simulink model "scheme1_analysis_aw"  (R2019b)
settings: Solver=ode4  StartTime=0.0  StopTime=30  FixedStep=0.1  RelTol=1e-3
values from neighbouring files (symbols this model uses):
  Kaw = 10    [solution.m]
  Kd = K(3)    [solution.m]
  Ki = K(1)    [solution.m]
  Kp = K(2)    [solution.m]
settings Model: Creator=biannic  LastModifiedBy=biannic
settings DataIOCC: ReturnWorkspaceOutputs=off

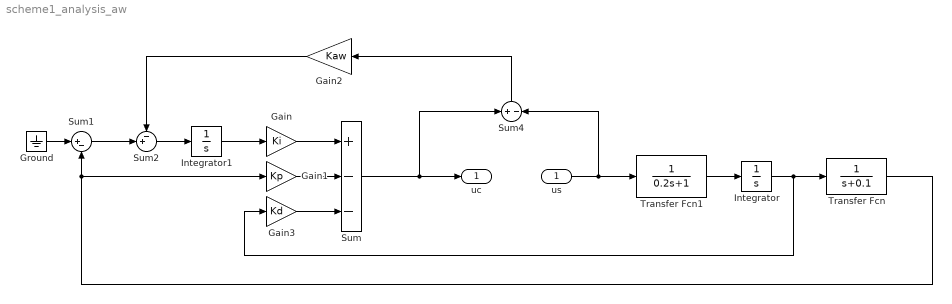
== system scheme1_analysis_aw ==
  us : Inport
  Gain : Gain  Gain=Ki
  Gain1 : Gain  Gain=Kp
  Gain2 : Gain  Gain=Kaw
  Gain3 : Gain  Gain=Kd
  Ground : Ground
  Integrator : Integrator
  Integrator1 : Integrator
  Sum : Sum  Inputs=+--
  Sum1 : Sum  Inputs=|+-
  Sum2 : Sum  Inputs=-+|
  Sum4 : Sum  Inputs=+|-
  Transfer Fcn : TransferFcn  Denominator=[1 0.1]
  Transfer Fcn1 : TransferFcn  Denominator=[0.2 1]
  uc : Outport
  wires:
  Ground/1 -> Sum1/1
  Sum/1 -> uc/1, Sum4/1
  us/1 -> Transfer Fcn1/1, Sum4/2
  Integrator/1 -> Gain3/1, Transfer Fcn/1
  Transfer Fcn/1 -> Gain1/1, Sum1/2
  Sum1/1 -> Sum2/2
  Sum2/1 -> Integrator1/1
  Sum4/1 -> Gain2/1
  Gain2/1 -> Sum2/1
  Transfer Fcn1/1 -> Integrator/1
  Gain3/1 -> Sum/3
  Gain1/1 -> Sum/2
  Gain/1 -> Sum/1
  Integrator1/1 -> Gain/1
